simulink model "aufgabe_2"  (R2017b)
settings: Solver=ode5  StartTime=0.0  StopTime=10.0e-3  FixedStep=1e-5  RelTol=1e-3
values from neighbouring files (symbols this model uses):
  f = logspace(2, 4, 100)    [aufgabe2.m]
settings Model: Creator=gurbuz  LastModifiedBy=gurbuz

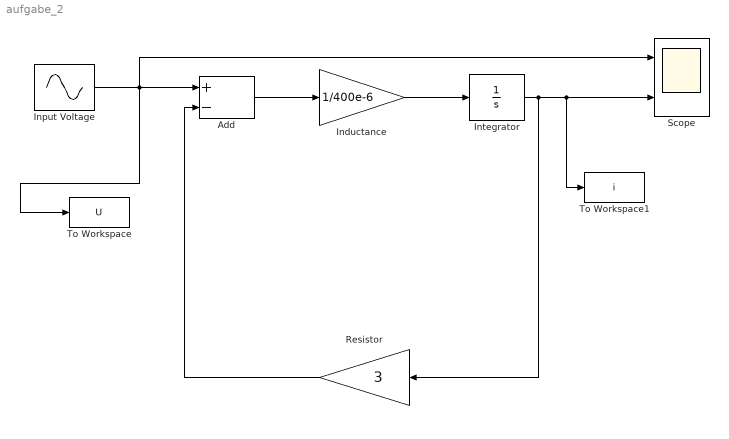
== system aufgabe_2 ==
  Add : Sum  Inputs=+-
  "Inductance " : Gain  Gain=1/400e-6
  "Input Voltage " : Sin  Amplitude=12  Frequency=f * 2 * pi  SampleTime=0
  Integrator : Integrator
  Resistor : Gain  Gain=3
  Scope : Scope  NumInputPorts=2
  To Workspace : ToWorkspace  VariableName=U  SampleTime=-1
      settings: Save2DSignal=2-D array (concatenate along first dimension)
  To Workspace1 : ToWorkspace  VariableName=i  SampleTime=-1
      settings: Save2DSignal=2-D array (concatenate along first dimension)
  wires:
  "Input Voltage "/1 -> To Workspace/1, Scope/1, Add/1
  Add/1 -> "Inductance "/1
  "Inductance "/1 -> Integrator/1
  Integrator/1 -> To Workspace1/1, Scope/2, Resistor/1
  Resistor/1 -> Add/2
